simulink subsystem "UserSCM"  (R2024b)
settings: Solver=VariableStepAuto  StartTime=0.0  StopTime=10.0  RelTol=1e-3
undefined symbols (not defined in the file or in its folder): Ts
settings Model: ModifiedByFormat=Kyle  Creator=Kyle  LastModifiedBy=Kyle

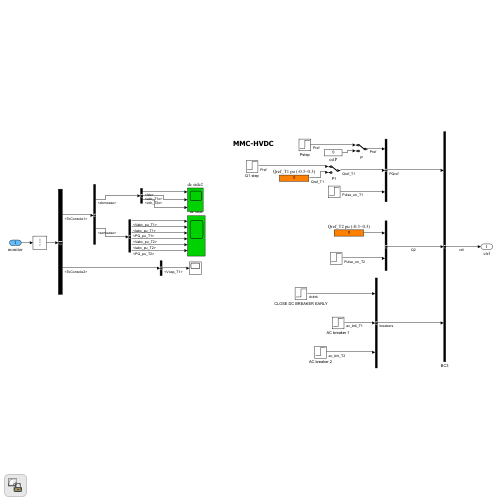
[thumbnail: Simulink's stored preview of the top-level diagram]
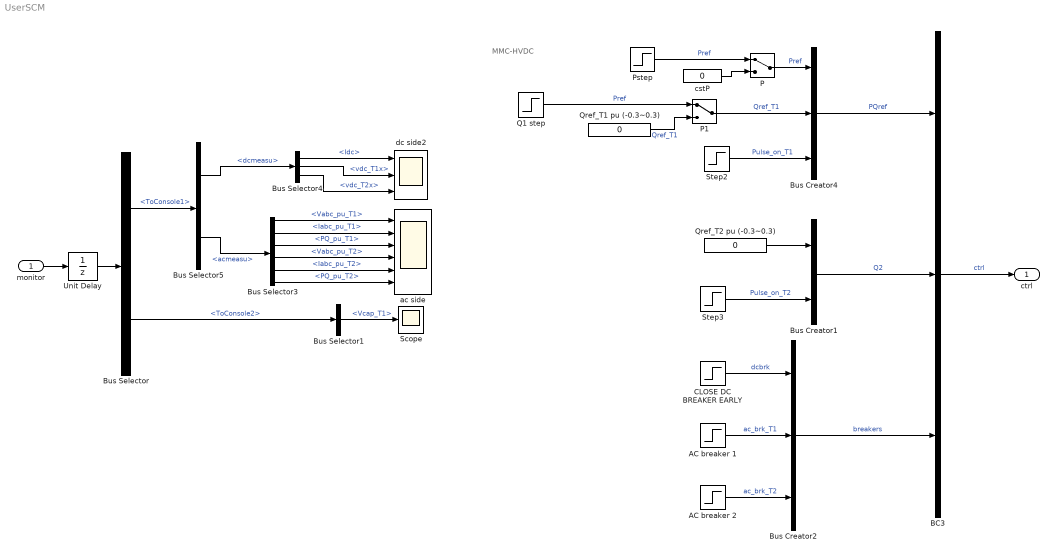
== system UserSCM ==
  note: MMC-HVDC
  monitor : Inport
  AC breaker 1 : Step  Time=0.4  SampleTime=Ts
  AC breaker 2 : Step  Time=0.45  SampleTime=Ts
  BC3 : BusCreator  Inputs=3  OutDataTypeStr=Bus: ctrl  NonVirtualBus=on
  Bus Creator1 : BusCreator  Inputs=2
  Bus Creator2 : BusCreator  Inputs=3
  Bus Creator4 : BusCreator  Inputs=3
  Bus Selector : BusSelector  OutputSignals=ToConsole1,ToConsole2
  Bus Selector1 : BusSelector  OutputSignals=Vcap_T1
  Bus Selector3 : BusSelector  OutputSignals=Vabc_pu_T1,Iabc_pu_T1,PQ_pu_T1,Vabc_pu_T2,Iabc_pu_T2,PQ_pu_T2
  Bus Selector4 : BusSelector  OutputSignals=Idc,Vdc_T1.vdc_T1x,Vdc_T2.vdc_T2x
  Bus Selector5 : BusSelector  OutputSignals=dcmeasu,acmeasu
  CLOSE DC BREAKER EARLY : Step  Time=0.1  SampleTime=Ts
  P : ManualSwitch
  P1 : ManualSwitch
  Pstep : Step  Time=0.9  After=0.4  SampleTime=Ts
  Q1 step : Step  Time=1.1  After=0.2  SampleTime=Ts
  Qref_T1 pu (-0.3~0.3) : Constant  Value=0
  Qref_T2 pu (-0.3~0.3) : Constant  Value=0
  Scope : Scope
  Step2 : Step  Time=0.6  SampleTime=Ts
  Step3 : Step  Time=0.6  SampleTime=Ts
  Unit Delay : UnitDelay  SampleTime=Ts  HasFrameUpgradeWarning=on
  ac side : Scope  NumInputPorts=6
  cstP : Constant  Value=0
  dc side2 : Scope  NumInputPorts=3
  ctrl : Outport  VectorParamsAs1DForOutWhenUnconnected=off
  wires:
  monitor/1 -> Unit Delay/1
  Bus Selector/1 -> Bus Selector5/1  "<ToConsole1>"
  Bus Selector/2 -> Bus Selector1/1  "<ToConsole2>"
  CLOSE DC BREAKER EARLY/1 -> Bus Creator2/1  "dcbrk"
  AC breaker 1/1 -> Bus Creator2/2  "ac_brk_T1"
  AC breaker 2/1 -> Bus Creator2/3  "ac_brk_T2"
  Bus Creator2/1 -> BC3/3  "breakers"
  Qref_T2 pu (-0.3~0.3)/1 -> Bus Creator1/1
  Step3/1 -> Bus Creator1/2  "Pulse_on_T2"
  Bus Creator1/1 -> BC3/2  "Q2"
  Bus Creator4/1 -> BC3/1  "PQref"
  Step2/1 -> Bus Creator4/3  "Pulse_on_T1"
  P/1 -> Bus Creator4/1  "Pref"
  Pstep/1 -> P/1  "Pref"
  cstP/1 -> P/2
  P1/1 -> Bus Creator4/2  "Qref_T1"
  Qref_T1 pu (-0.3~0.3)/1 -> P1/2  "Qref_T1"
  Q1 step/1 -> P1/1  "Pref"
  BC3/1 -> ctrl/1  "ctrl"
  Unit Delay/1 -> Bus Selector/1
  Bus Selector1/1 -> Scope/1  "<Vcap_T1>"
  Bus Selector4/3 -> dc side2/3  "<vdc_T2x>"
  Bus Selector4/2 -> dc side2/2  "<vdc_T1x>"
  Bus Selector4/1 -> dc side2/1  "<Idc>"
  Bus Selector5/2 -> Bus Selector3/1  "<acmeasu>"
  Bus Selector5/1 -> Bus Selector4/1  "<dcmeasu>"
  Bus Selector3/6 -> ac side/6  "<PQ_pu_T2>"
  Bus Selector3/5 -> ac side/5  "<Iabc_pu_T2>"
  Bus Selector3/4 -> ac side/4  "<Vabc_pu_T2>"
  Bus Selector3/3 -> ac side/3  "<PQ_pu_T1>"
  Bus Selector3/2 -> ac side/2  "<Iabc_pu_T1>"
  Bus Selector3/1 -> ac side/1  "<Vabc_pu_T1>"
